simulink model "KukaSimModel"  (R2021a)
settings: Solver=VariableStepAuto  StartTime=0.0  StopTime=20  FixedStep=0.01  RelTol=1e-3
PreLoadFcn:
  | TP_TASK_SPACE = Simulink.Variant('TP_MODE==1');
  | TP_JOINT_SPACE = Simulink.Variant('TP_MODE==2');
InitFcn:
  | if TP_MODE == 1
  |     %pass
  |     return;
  | end
  | jointWaypoints = zeros(6, size(waypointsStruct.waypoints, 2));
  | for i=1:size(waypointsStruct.waypoints, 2)
  |     jointWaypoints(:, i) = solver.solveInverseKinematics(dhParametersStruct, waypointsStruct.waypoints(:, i));
  | end
undefined symbols (not defined in the file): dhParametersStruct, dt_FixedStep, dynamicParametersStruct, q1, q2, q3, q4, q5, q6, waypointsStruct
libraries: lib_Solver x5
settings Model: Creator=chiar  LastModifiedBy=chiar
settings OptimizationCC: BlockReduction=off  DefaultParameterBehavior=Inlined  BufferReuse=off
settings GRTTargetCC: RTWCAPISignals=on  RTWCAPIParams=on

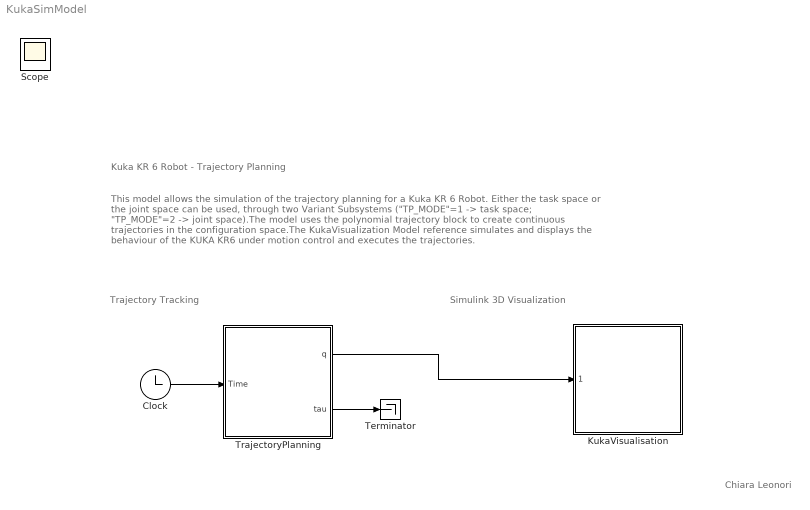
== system KukaSimModel ==
  note: Chiara Leonori
  note: Trajectory Tracking
  note: Simulink 3D Visualization
  note: This model allows the simulation of the trajectory planning for a Kuka KR 6 Robot. Either the task space or the joint space can be used, through two Variant Subsystems ("TP_MODE"=1 -> task space; "TP_MODE"=2 -> joint space).The model uses the polynomial trajectory block to create continuous trajectories in the configuration space.The KukaVisualization Model reference simulates and displays the behaviour of the KUKA KR6 under motion control and executes the trajectories.
  note: Kuka KR 6 Robot - Trajectory Planning
  Clock : Clock
  KukaVisualisation : Subsystem  ReferencedSubsystem=KukaVisualisationModel
  Terminator : Terminator
  TrajectoryPlanning : Subsystem  Variant=on
  Scope : Scope
  wires:
  TrajectoryPlanning/1(q) -> KukaVisualisation/1
  Clock/1 -> TrajectoryPlanning/1(Time)
  TrajectoryPlanning/2(tau) -> Terminator/1

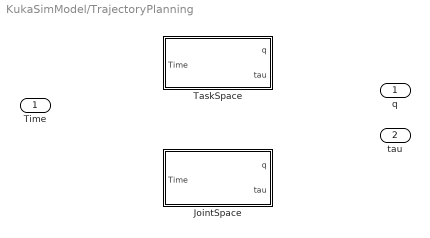
== system KukaSimModel/TrajectoryPlanning ==
  Time : Inport
  JointSpace : Subsystem  VariantControl=TP_MODE == 2
  TaskSpace : Subsystem  VariantControl=TP_MODE == 1
  q : Outport  OutDataTypeStr=Bus: Bus_q
  tau : Outport  Port=2  OutDataTypeStr=double

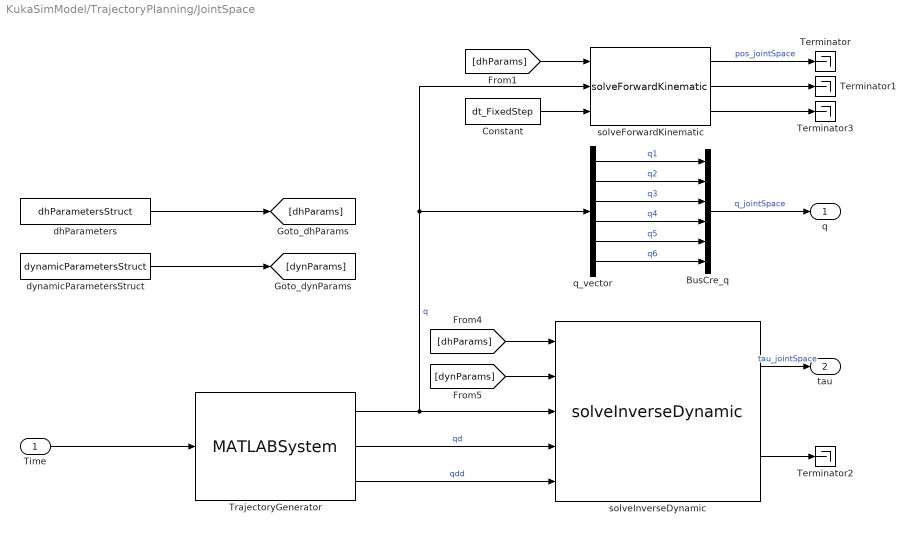
== system KukaSimModel/TrajectoryPlanning/JointSpace ==
  Time : Inport
  BusCre_q : BusCreator  Inputs=q1,q2,q3,q4,q5,q6  OutDataTypeStr=Bus: Bus_q
  Constant : Constant  Value=dt_FixedStep
  Terminator{,1..3} (4 alike) : Terminator
  TrajectoryGenerator : MATLABSystem  System=core.TrajectoryGenerator  Method=Quintic Polynomial  Waypoints=jointWaypoints  Timepoints=waypointsStruct.times  Velocities=zeros(6, size(waypointsStruct.waypoints, 2))  Accelerations=zeros(6, size(waypointsStruct.waypoints, 2))  SimulateUsing=Interpreted execution
      mask Type: core.TrajectoryGenerator
      mask Display:
      | image('srcs\simulink\blockicons\polynomial-icon-big.jpg');
      | port_label('input',1,'t');
      | port_label('output',1,'q_out');
      | port_label('output',2,'qd_out');
      | port_label('output',3,'qdd_out');
  dhParameters : Constant  Value=dhParametersStruct  OutDataTypeStr=Bus: Bus_dhParameter
  dynamicParametersStruct : Constant  Value=dynamicParametersStruct  OutDataTypeStr=Bus: Bus_dynamicsParameter
  q_vector : Demux  Outputs=6
  solveForwardKinematic : lib_Solver/solveForwardKinematic  SystemSampleTime=-1  VariantActivationTime=update diagram  Latency=0  AutoFrameSizeCalculation=off
      settings: SourceProductBaseCode=SL
  solveInverseDynamic : lib_Solver/solveInverseDynamic  SystemSampleTime=-1  VariantActivationTime=update diagram  Latency=0  AutoFrameSizeCalculation=off
      settings: SourceProductBaseCode=SL
  q : Outport  OutDataTypeStr=Bus: Bus_q
  tau : Outport  Port=2  OutDataTypeStr=double
  wires:
  Time/1 -> TrajectoryGenerator/1
  [dynParams] -> solveInverseDynamic/2
  [dhParams] -> solveInverseDynamic/1
  TrajectoryGenerator/2 -> solveInverseDynamic/4  "qd"
  TrajectoryGenerator/3 -> solveInverseDynamic/5  "qdd"
  solveInverseDynamic/1 -> tau/1  "tau_jointSpace"
  q_vector/6 -> BusCre_q/6  "q6"
  q_vector/1 -> BusCre_q/1  "q1"
  q_vector/2 -> BusCre_q/2  "q2"
  q_vector/3 -> BusCre_q/3  "q3"
  q_vector/5 -> BusCre_q/5  "q5"
  q_vector/4 -> BusCre_q/4  "q4"
  TrajectoryGenerator/1 -> solveInverseDynamic/3, solveForwardKinematic/2, q_vector/1  "q"
  BusCre_q/1 -> q/1  "q_jointSpace"
  solveInverseDynamic/2 -> Terminator2/1
  dhParameters/1 -> [dhParams]
  dynamicParametersStruct/1 -> [dynParams]
  [dhParams] -> solveForwardKinematic/1
  Constant/1 -> solveForwardKinematic/3
  solveForwardKinematic/1 -> Terminator/1  "pos_jointSpace"
  solveForwardKinematic/2 -> Terminator1/1
  solveForwardKinematic/3 -> Terminator3/1

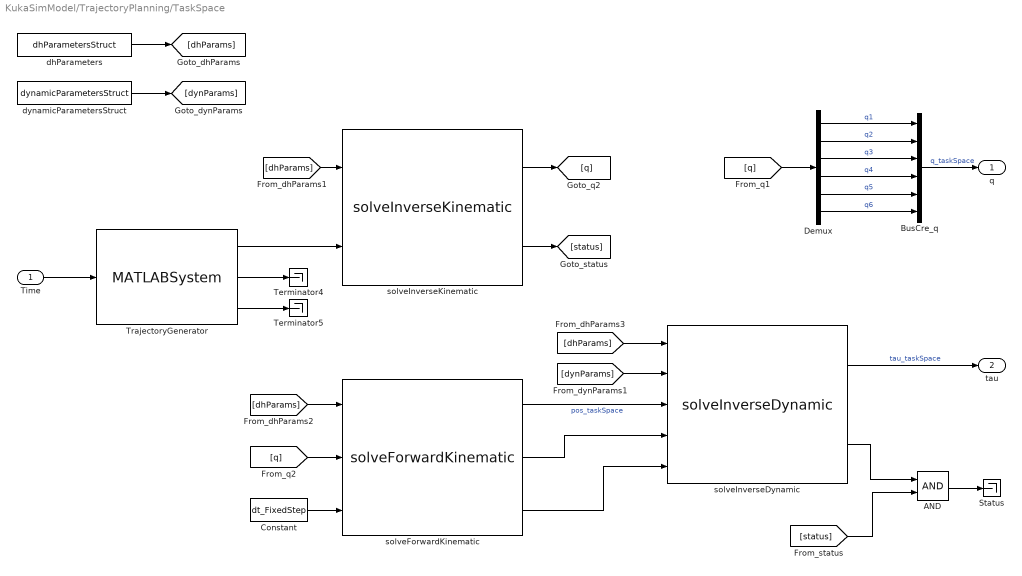
== system KukaSimModel/TrajectoryPlanning/TaskSpace ==
  Time : Inport
  AND : Logic  AllPortsSameDT=off  OutDataTypeStr=boolean
  BusCre_q : BusCreator  Inputs=q1,q2,q3,q4,q5,q6  OutDataTypeStr=Bus: Bus_q
  Constant : Constant  Value=dt_FixedStep  OutDataTypeStr=double
  Demux : Demux  Outputs=6
  Status : Terminator
  Terminator4 : Terminator
  Terminator5 : Terminator
  TrajectoryGenerator : MATLABSystem  System=core.TrajectoryGenerator  Method=Quintic Polynomial  Waypoints=waypointsStruct.waypoints  Timepoints=waypointsStruct.times  Velocities=waypointsStruct.velocities  Accelerations=waypointsStruct.accelerations  SimulateUsing=Interpreted execution
      mask Type: core.TrajectoryGenerator
      mask Display:
      | image('srcs\simulink\blockicons\polynomial-icon-big.jpg');
      | port_label('input',1,'t');
      | port_label('output',1,'q_out');
      | port_label('output',2,'qd_out');
      | port_label('output',3,'qdd_out');
  dhParameters : Constant  Value=dhParametersStruct  OutDataTypeStr=Bus: Bus_dhParameter
  dynamicParametersStruct : Constant  Value=dynamicParametersStruct  OutDataTypeStr=Bus: Bus_dynamicsParameter
  solveForwardKinematic : lib_Solver/solveForwardKinematic  SystemSampleTime=-1  VariantActivationTime=update diagram  Latency=0  AutoFrameSizeCalculation=off
      settings: SourceProductBaseCode=SL
  solveInverseDynamic : lib_Solver/solveInverseDynamic  SystemSampleTime=-1  VariantActivationTime=update diagram  Latency=0  AutoFrameSizeCalculation=off
      settings: SourceProductBaseCode=SL
  solveInverseKinematic : lib_Solver/solveInverseKinematic  SystemSampleTime=-1  VariantActivationTime=update diagram  Latency=0  AutoFrameSizeCalculation=off
      settings: SourceProductBaseCode=SL
  q : Outport  OutDataTypeStr=Bus: Bus_q
  tau : Outport  Port=2  OutDataTypeStr=double
  wires:
  Time/1 -> TrajectoryGenerator/1
  solveInverseDynamic/1 -> tau/1  "tau_taskSpace"
  TrajectoryGenerator/2 -> Terminator4/1
  TrajectoryGenerator/3 -> Terminator5/1
  Demux/1 -> BusCre_q/1  "q1"
  Demux/2 -> BusCre_q/2  "q2"
  Demux/3 -> BusCre_q/3  "q3"
  Demux/4 -> BusCre_q/4  "q4"
  Demux/5 -> BusCre_q/5  "q5"
  Demux/6 -> BusCre_q/6  "q6"
  BusCre_q/1 -> q/1  "q_taskSpace"
  TrajectoryGenerator/1 -> solveInverseKinematic/2
  solveInverseDynamic/2 -> AND/1
  AND/1 -> Status/1
  Constant/1 -> solveForwardKinematic/3
  [status] -> AND/2
  [q] -> Demux/1
  [q] -> solveForwardKinematic/2
  solveInverseKinematic/1 -> [q]
  solveInverseKinematic/2 -> [status]
  solveForwardKinematic/1 -> solveInverseDynamic/3  "pos_taskSpace"
  solveForwardKinematic/2 -> solveInverseDynamic/4
  solveForwardKinematic/3 -> solveInverseDynamic/5
  dhParameters/1 -> [dhParams]
  [dhParams] -> solveForwardKinematic/1
  [dhParams] -> solveInverseDynamic/1
  [dynParams] -> solveInverseDynamic/2
  dynamicParametersStruct/1 -> [dynParams]
  [dhParams] -> solveInverseKinematic/1
